simulink model "full_TriPed_simulation"  (R2021a)
settings: Solver=daessc  StartTime=0.0  StopTime=10  RelTol=1e-3
undefined symbols (not defined in the file or in its folder): X, Y, Z
libraries: sm_lib x8, TripedLibrary x6, simulink x5, spsFirstOrderFilterLib x4, nesl_utility x4
settings Model: Creator=jan-b  LastModifiedBy=maxde

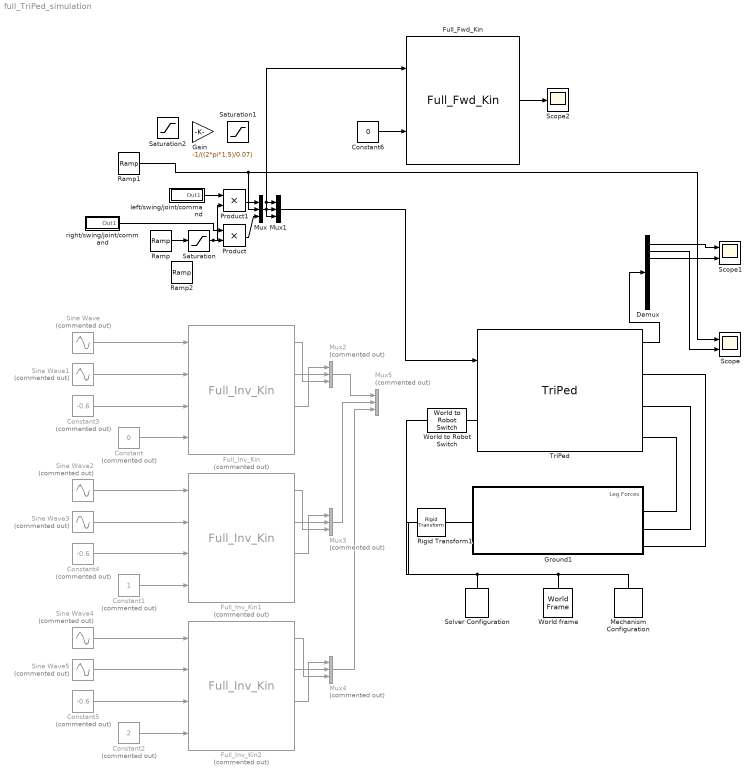
== system full_TriPed_simulation ==
  Constant : Constant  Commented=on  Value=0
  Constant1 : Constant  Commented=on
  Constant2 : Constant  Commented=on  Value=2
  Constant3 : Constant  Commented=on  Value=-0.6
  Constant4 : Constant  Commented=on  Value=-0.6
  Constant5 : Constant  Commented=on  Value=-0.6
  Constant6 : Constant  Value=0
  Demux : Demux  Outputs=9
  Full_Fwd_Kin : TripedLibrary/Kinematic Utils/Full Model kinematics/Full_Fwd_Kin  SystemSampleTime=-1  VariantActivationTime=update diagram  Latency=0  AutoFrameSizeCalculation=off
      settings: SourceProductName=TriPed Library
  Full_Inv_Kin : TripedLibrary/Kinematic Utils/Full Model kinematics/Full_Inv_Kin  Commented=on  SystemSampleTime=-1  VariantActivationTime=update diagram  Latency=0  AutoFrameSizeCalculation=off
      settings: SourceProductName=TriPed Library
  Full_Inv_Kin1 : TripedLibrary/Kinematic Utils/Full Model kinematics/Full_Inv_Kin  Commented=on  SystemSampleTime=-1  VariantActivationTime=update diagram  Latency=0  AutoFrameSizeCalculation=off
      settings: SourceProductName=TriPed Library
  Full_Inv_Kin2 : TripedLibrary/Kinematic Utils/Full Model kinematics/Full_Inv_Kin  Commented=on  SystemSampleTime=-1  VariantActivationTime=update diagram  Latency=0  AutoFrameSizeCalculation=off
      settings: SourceProductName=TriPed Library
  Gain : Gain  Gain=-1/((2*pi*1.5)/0.07)
  Ground1 : Subsystem
  Mechanism Configuration : sm_lib/Utilities/Mechanism Configuration  UniformGravity=Constant  GravityVector=[0 0 -9.80665]  GravityVectorUnits=m/s^2  GravityUnits=m/s^2  LinearizationDelta=0.001  JointModeTransitionNonlinearIterations=2
  Mux : Mux  Inputs=3
  Mux1 : Mux  Inputs=3
  Mux{2..5} (4 alike) : Mux  Commented=on  Inputs=3
  Product : Product
  Product1 : Product
  Ramp : simulink/Sources/Ramp  slope=1  start=0  InitialOutput=0
  Ramp1 : simulink/Sources/Ramp  slope=0.1  start=0  InitialOutput=0
  Ramp2 : simulink/Sources/Ramp  slope=-0.3  start=0  InitialOutput=0
  Rigid Transform1 : sm_lib/Frames and Transforms/Rigid Transform  TranslationMethod=Cartesian  TranslationStandardOffset=-0.7  TranslationLengthUnit=m  TranslationStandardAxis=+Z  TranslationCartesianOffset="[1.5  0 -0.7]"  TranslationROffset=0  TranslationROffsetUnits=m  TranslationZOffset=0  TranslationZOffsetUnits=m  TranslationThetaOffset=0  TranslationThetaOffsetUnits=deg  RotationMethod=None  RotationAngleUnits=deg  RotationStandardAxis=+Z  RotationAngle=0.0  RotationArbitraryAxis=[0 0 1]  FollAlignAxisA=+X  BaseAlignAxisA=+Y  FollAlignAxisB=+Y  BaseAlignAxisB=+Z  RotationSequenceAxes=FollowerAxes  RotationSequence=XYX  RotationSequenceAngles=[0 0 0]  RotationSequenceAnglesUnits=deg  RotationMatrix=[1 0 0; 0 1 0; 0 0 1]
  Saturation : Saturate  UpperLimit=1  LowerLimit=0
  Saturation1 : Saturate  UpperLimit=1  LowerLimit=0
  Saturation2 : Saturate  LowerLimit=0
  Scope : Scope  NumInputPorts=2
  Scope1 : Scope  NumInputPorts=2
  Scope2 : Scope
  Sine Wave : Sin  Commented=on  Amplitude=0.2  Bias=0.3  SampleTime=0
  Sine Wave1 : Sin  Commented=on  Amplitude=0.2  Bias=0.3  Phase=pi/2  SampleTime=0
  Sine Wave2 : Sin  Commented=on  Amplitude=0.2  Bias=0.3  SampleTime=0
  Sine Wave3 : Sin  Commented=on  Amplitude=0.2  Bias=0.3  Phase=pi/2  SampleTime=0
  Sine Wave4 : Sin  Commented=on  Amplitude=0.2  Bias=0.3  SampleTime=0
  Sine Wave5 : Sin  Commented=on  Amplitude=0.2  Bias=0.3  Phase=pi/2  SampleTime=0
  Solver Configuration : nesl_utility/Solver Configuration  PhysicalDomain=network_engine_domain  SubClassName=solver  LeftPortType=input  RightPortType=generic  Tones=[]  Harmonics=[]  SimulateNoise=off  Profile=off  UseLocalSampling=off  EnableSwitchedLinearOptims=on  FrequencyDomain=off  UseCCode=off  RelTol=0.001  AbsTol=1e-06  MinStep=1e-09  ToWorkspace=off  RevertToSquareIcSolve=off  NumHomotopyIterations=100  PhasorMode=off  PhasorModeNumHarmonics=1  DoDC=off  ResidualTolerance=1e-06  UseLocalSolver=off  LocalSolverChoice=NE_BACKWARD_EULER_ADVANCER  LocalSolverSampleTime=0.001  DoFixedCost=off  MaxNonlinIter=3  MaxModeIter=2  ComputeImpulses=off  ImpulseIterations=2  LinearAlgebra=Sparse  EquationFormulation=NE_TIME_EF  DelaysMemoryBudget=1024  AutomaticFiltering=on  FilteringTimeConstant=0.001  PartitionStorageMethod=AS_NEEDED  PartitionMemoryBudget=1024  PartitionMethod=FAST
  TriPed : TripedLibrary/Full Model/TriPed  SystemSampleTime=-1  VariantActivationTime=update diagram  Latency=0  AutoFrameSizeCalculation=off
      settings: SourceProductName=TriPed Library
  World frame : sm_lib/Frames and Transforms/World Frame
  World to Robot Switch : TripedLibrary/Environment/World to Robot Switch  SystemSampleTime=-1  LabelModeActiveChoice=Choice_2  VariantActivationTime=update diagram  Latency=0  AutoFrameSizeCalculation=off
      settings: SourceProductName=TriPed Library
  left/swing/joint/command : Subsystem
  right/swing/joint/command : Subsystem
  wires:
  right/swing/joint/command/1(Out1) -> Product/1
  Mux/1 -> Full_Fwd_Kin/1, Mux1/1, Mux1/3, Mux1/2
  TriPed/1 -> Demux/1
  left/swing/joint/command/1(Out1) -> Product1/1
  Ramp/1 -> Saturation/1
  Saturation/1 -> Product1/2, Product/2
  Product/1 -> Mux/3
  Ramp1/1 -> Mux/2, Scope/1
  Demux/2 -> Scope/2
  Demux/1 -> Scope1/1
  Demux/3 -> Scope1/2
  Product1/1 -> Mux/1
  Constant/1 -> Full_Inv_Kin/4
  Full_Inv_Kin/1 -> Mux2/3
  Full_Inv_Kin/3 -> Mux2/1
  Full_Inv_Kin/2 -> Mux2/2
  Full_Inv_Kin1/2 -> Mux3/2
  Full_Inv_Kin1/1 -> Mux3/3
  Constant1/1 -> Full_Inv_Kin1/4
  Full_Inv_Kin1/3 -> Mux3/1
  Full_Inv_Kin2/2 -> Mux4/2
  Full_Inv_Kin2/1 -> Mux4/3
  Constant2/1 -> Full_Inv_Kin2/4
  Full_Inv_Kin2/3 -> Mux4/1
  Mux2/1 -> Mux5/1
  Mux3/1 -> Mux5/2
  Mux4/1 -> Mux5/3
  Sine Wave/1 -> Full_Inv_Kin/1
  Sine Wave1/1 -> Full_Inv_Kin/2
  Constant3/1 -> Full_Inv_Kin/3
  Sine Wave2/1 -> Full_Inv_Kin1/1
  Sine Wave3/1 -> Full_Inv_Kin1/2
  Constant4/1 -> Full_Inv_Kin1/3
  Sine Wave4/1 -> Full_Inv_Kin2/1
  Sine Wave5/1 -> Full_Inv_Kin2/2
  Constant5/1 -> Full_Inv_Kin2/3
  Mux1/1 -> TriPed/1
  Constant6/1 -> Full_Fwd_Kin/2
  Full_Fwd_Kin/1 -> Scope2/1
  connections:
  World frame/RConn1 -- World to Robot Switch/LConn1 -- Rigid Transform1/LConn1 -- Solver Configuration/RConn1 -- Mechanism Configuration/RConn1
  Ground1/RConn2 -- TriPed/RConn2
  Ground1/RConn1 -- TriPed/RConn3
  Ground1/RConn3 -- TriPed/RConn1
  Rigid Transform1/RConn1 -- Ground1/LConn1
  World to Robot Switch/RConn1 -- TriPed/LConn1

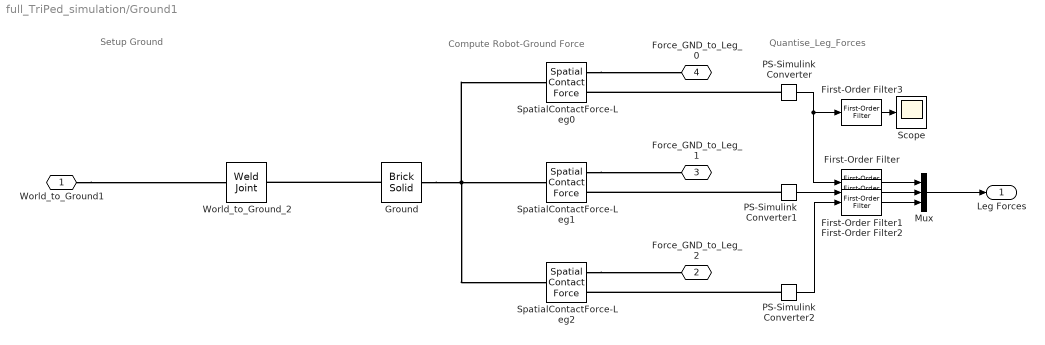
== system full_TriPed_simulation/Ground1 ==
  note: Setup Ground
  note: Compute Robot-Ground Force
  note: Quantise_Leg_Forces
  First-Order Filter : spsFirstOrderFilterLib/First-Order Filter  FilterType=Lowpass  Tc=1/30  Ts=0  Initialize=on  Vac_Init=[0, 0, 60]  Vdc_Init=0  PlotResponse=off  FreqRange="[0,  200,  1]"
  First-Order Filter1 : spsFirstOrderFilterLib/First-Order Filter  FilterType=Lowpass  Tc=1/30  Ts=0  Initialize=on  Vac_Init=[0, 0, 60]  Vdc_Init=0  PlotResponse=off  FreqRange="[0,  200,  1]"
  First-Order Filter2 : spsFirstOrderFilterLib/First-Order Filter  FilterType=Lowpass  Tc=1/30  Ts=0  Initialize=on  Vac_Init=[0, 0, 60]  Vdc_Init=0  PlotResponse=off  FreqRange="[0,  200,  1]"
  First-Order Filter3 : spsFirstOrderFilterLib/First-Order Filter  FilterType=Lowpass  Tc=1/5  Ts=0  Initialize=on  Vac_Init=[0, 0, 60]  Vdc_Init=0  PlotResponse=off  FreqRange="[0,  200,  1]"
  Ground : sm_lib/Body Elements/Brick Solid  GraphicAmbientColor=[0.15 0.15 0.15 1.0]  BasedOnType=Density  BrickDimensions=[5 5 0.1]  BrickDimensionUnits=m  CenterOfMass=[0 0 0]  CenterOfMassUnits=m  GraphicDiffuseColor=[0.4 0.4 0.4]  Density=1000  DensityUnits=kg/m^3  DoExposeReferenceFrame=on  GraphicEmissiveColor=[0.0 0.0 0.0 1.0]  ExportEntireGeometry=on  SerializedFrames=<Frames/>  MarkerShape=Sphere  MarkerSize=10  GraphicType=FromGeometry  InertiaType=CalculateFromGeometry  Mass=1  MassUnits=kg  MomentsOfInertia=[1 1 1]  MomentsOfInertiaUnits=kg*m^2  GraphicOpacity=0.8  ProductsOfInertia=[0 0 0]  ProductsOfInertiaUnits=kg*m^2  GraphicShininess=75  GraphicSpecularColor=[0.5 0.5 0.5 1.0]  GraphicVisPropType=SimpleVisualProperties
  Mux : Mux  Inputs=3
  PS-Simulink Converter : nesl_utility/PS-Simulink Converter  PhysicalDomain=network_engine_domain  SubClassName=ps_output  LeftPortType=input  RightPortType=output  PseudoPeriodic=off  Frequencies=[]  Unit=inherit  AffineConversion=off
  PS-Simulink Converter1 : nesl_utility/PS-Simulink Converter  PhysicalDomain=network_engine_domain  SubClassName=ps_output  LeftPortType=input  RightPortType=output  PseudoPeriodic=off  Frequencies=[]  Unit=inherit  AffineConversion=off
  PS-Simulink Converter2 : nesl_utility/PS-Simulink Converter  PhysicalDomain=network_engine_domain  SubClassName=ps_output  LeftPortType=input  RightPortType=output  PseudoPeriodic=off  Frequencies=[]  Unit=inherit  AffineConversion=off
  Scope : Scope
  SpatialContactForce-Leg0 : sm_lib/Forces and Torques/Spatial Contact Force  CoefficientOfDynamicFriction=0.6  CoefficientOfStaticFriction=1  SenseContactBaseRotation=off  SenseContactBaseTranslation=off  NormalDamping=10^3  NormalDampingUnits=N/(m/s)  SenseContactFollowerRotation=off  SenseContactFollowerTranslation=off  SenseContactSignal=off  NormalStiffness=30000  NormalStiffnessUnits=N/m  FrictionalCriticalVelocity=1e-2  FrictionalCriticalVelocityUnits=m/s  ZeroCrossDetectContactStartAndEnd=on  FrictionType=SmoothStickSlip  SenseFrictionalForceMagnitude=off  SenseNormalForceMagnitude=on  NormalForceType=SmoothSpringDamper  SenseNormalVelocity=off  SenseSeparationDistance=off  SenseTangentialVelocity=off  SenseTangentialVelocityMagnitude=off  NormalTransitionRegionWidth=1e-3  NormalTransitionRegionWidthUnits=m
  SpatialContactForce-Leg1 : sm_lib/Forces and Torques/Spatial Contact Force  CoefficientOfDynamicFriction=0.6  CoefficientOfStaticFriction=1  SenseContactBaseRotation=off  SenseContactBaseTranslation=off  NormalDamping=10^3  NormalDampingUnits=N/(m/s)  SenseContactFollowerRotation=off  SenseContactFollowerTranslation=off  SenseContactSignal=off  NormalStiffness=30000  NormalStiffnessUnits=N/m  FrictionalCriticalVelocity=1e-2  FrictionalCriticalVelocityUnits=m/s  ZeroCrossDetectContactStartAndEnd=on  FrictionType=SmoothStickSlip  SenseFrictionalForceMagnitude=off  SenseNormalForceMagnitude=on  NormalForceType=SmoothSpringDamper  SenseNormalVelocity=off  SenseSeparationDistance=off  SenseTangentialVelocity=off  SenseTangentialVelocityMagnitude=off  NormalTransitionRegionWidth=1e-3  NormalTransitionRegionWidthUnits=m
  SpatialContactForce-Leg2 : sm_lib/Forces and Torques/Spatial Contact Force  CoefficientOfDynamicFriction=0.6  CoefficientOfStaticFriction=1  SenseContactBaseRotation=off  SenseContactBaseTranslation=off  NormalDamping=10^3  NormalDampingUnits=N/(m/s)  SenseContactFollowerRotation=off  SenseContactFollowerTranslation=off  SenseContactSignal=off  NormalStiffness=30000  NormalStiffnessUnits=N/m  FrictionalCriticalVelocity=1e-2  FrictionalCriticalVelocityUnits=m/s  ZeroCrossDetectContactStartAndEnd=on  FrictionType=SmoothStickSlip  SenseFrictionalForceMagnitude=off  SenseNormalForceMagnitude=on  NormalForceType=SmoothSpringDamper  SenseNormalVelocity=off  SenseSeparationDistance=off  SenseTangentialVelocity=off  SenseTangentialVelocityMagnitude=off  NormalTransitionRegionWidth=1e-3  NormalTransitionRegionWidthUnits=m
  World_to_Ground_2 : sm_lib/Joints/Weld Joint  JointMode=Normal  SenseConstraintForce=off  SenseConstraintForceX=off  SenseConstraintForceY=off  SenseConstraintForceZ=off  SenseConstraintTorque=off  SenseConstraintTorqueX=off  SenseConstraintTorqueY=off  SenseConstraintTorqueZ=off  SenseTotalForce=off  SenseTotalForceX=off  SenseTotalForceY=off  SenseTotalForceZ=off  SenseTotalTorque=off  SenseTotalTorqueX=off  SenseTotalTorqueY=off  SenseTotalTorqueZ=off  CompositeWrenchDir=FollowerOnBase  CompositeWrenchFrame=BaseFrame
  World_to_Ground1 : PMIOPort  Side=Left
  Force_GND_to_Leg_2 : PMIOPort  Port=2  Side=Right
  Force_GND_to_Leg_1 : PMIOPort  Port=3  Side=Right
  Force_GND_to_Leg_0 : PMIOPort  Port=4  Side=Right
  Leg Forces : Outport
  wires:
  PS-Simulink Converter/1 -> First-Order Filter3/1, First-Order Filter/1
  PS-Simulink Converter1/1 -> First-Order Filter1/1
  PS-Simulink Converter2/1 -> First-Order Filter2/1
  Mux/1 -> Leg Forces/1
  First-Order Filter/1 -> Mux/1
  First-Order Filter1/1 -> Mux/2
  First-Order Filter2/1 -> Mux/3
  First-Order Filter3/1 -> Scope/1
  connections:
  Ground/RConn1 -- World_to_Ground_2/RConn1
  Ground/LConn1 -- SpatialContactForce-Leg0/LConn1 -- SpatialContactForce-Leg1/LConn1 -- SpatialContactForce-Leg2/LConn1
  SpatialContactForce-Leg1/RConn1 -- Force_GND_to_Leg_1/RConn1
  SpatialContactForce-Leg2/RConn1 -- Force_GND_to_Leg_2/RConn1
  SpatialContactForce-Leg0/RConn1 -- Force_GND_to_Leg_0/RConn1
  World_to_Ground1/RConn1 -- World_to_Ground_2/LConn1
  PS-Simulink Converter1/LConn1 -- SpatialContactForce-Leg1/RConn2
  PS-Simulink Converter2/LConn1 -- SpatialContactForce-Leg2/RConn2
  PS-Simulink Converter/LConn1 -- SpatialContactForce-Leg0/RConn2

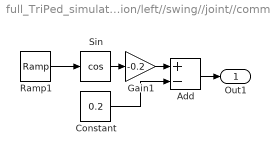
== system full_TriPed_simulation/left//swing//joint//command ==
  Add : Sum  Inputs=+-
  Constant : Constant  Value=0.2
  Gain1 : Gain  Gain=-0.2
  Ramp1 : simulink/Sources/Ramp  slope=0.8  start=0  InitialOutput=0
  Sin : Trigonometry  Operator=cos
  Out1 : Outport
  wires:
  Gain1/1 -> Add/1
  Sin/1 -> Gain1/1
  Ramp1/1 -> Sin/1
  Add/1 -> Out1/1
  Constant/1 -> Add/2

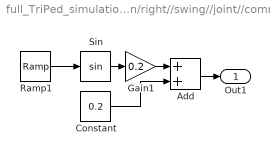
== system full_TriPed_simulation/right//swing//joint//command ==
  Add : Sum
  Constant : Constant  Value=0.2
  Gain1 : Gain  Gain=0.2
  Ramp1 : simulink/Sources/Ramp  slope=0.8  start=0  InitialOutput=0
  Sin : Trigonometry
  Out1 : Outport
  wires:
  Gain1/1 -> Add/1
  Sin/1 -> Gain1/1
  Ramp1/1 -> Sin/1
  Add/1 -> Out1/1
  Constant/1 -> Add/2
